simulink model "pidControllerAltitudeSystem"  (R2023b)
settings: Solver=VariableStepAuto  StartTime=0.0  StopTime=10  RelTol=1e-3
settings Model: Creator=mvhod  LastModifiedBy=mvhod

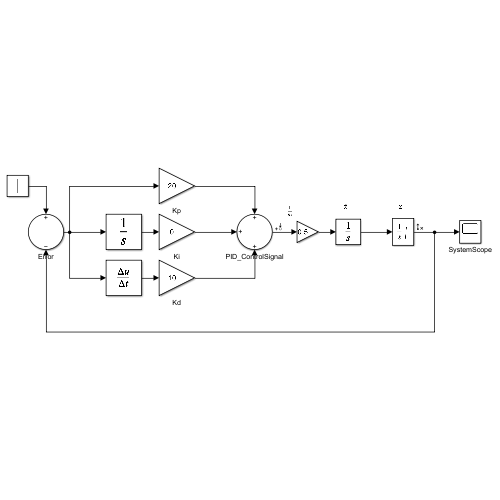
[thumbnail: Simulink's stored preview of the top-level diagram]
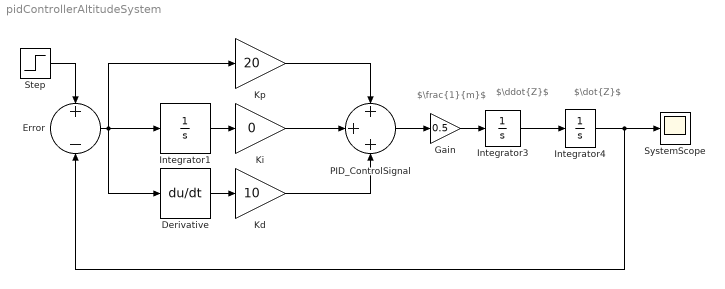
== system pidControllerAltitudeSystem ==
  note: $\ddot{Z}$
  note: $\frac{1}{m}$
  note: $\dot{Z}$
  Derivative : Derivative
  Error : Sum  Inputs=+-
  Gain : Gain  Gain=0.5
  Integrator1 : Integrator
  Integrator3 : Integrator
  Integrator4 : Integrator  LimitOutput=on  LowerSaturationLimit=0
  Kd : Gain  Gain=10
  Ki : Gain  Gain=0
  Kp : Gain  Gain=20
  PID_ControlSignal : Sum  Inputs=+++
  Step : Step  Time=0  SampleTime=0
  SystemScope : Scope
  wires:
  Integrator1/1 -> Ki/1
  Error/1 -> Integrator1/1, Derivative/1, Kp/1
  Derivative/1 -> Kd/1
  Kp/1 -> PID_ControlSignal/1
  PID_ControlSignal/1 -> Gain/1
  Ki/1 -> PID_ControlSignal/2
  Kd/1 -> PID_ControlSignal/3
  Integrator3/1 -> Integrator4/1
  Gain/1 -> Integrator3/1
  Step/1 -> Error/1
  Integrator4/1 -> SystemScope/1, Error/2
